simulink model "rotation"  (Simulink 7.0)
settings: Solver=ode45  SolverMode=SingleTasking  StartTime=0.0  StopTime=inf  RelTol=1e-3
values from neighbouring files (symbols this model uses):
  blk = 10    [rotation_init.m]
  col_delx_ws = ceil(col_delx*2^20)    [rotation_init.m]
  col_dely_ws = ceil(col_dely*2^20)    [rotation_init.m]
  fps = 1/(rows*(cols+3*blk))    [rotation_init.m]
  row_delx_ws = ceil(row_delx*2^20)*2    [rotation_init.m]
  row_dely_ws = ceil(row_dely*2^20)*2    [rotation_init.m]
  xstart_init_ws = ceil(xstart_init*2^20)    [rotation_init.m]
  ystart_init_ws = ceil(ystart_init*2^20)    [rotation_init.m]
undefined symbols (not defined in the file or in its folder): cols, rows
libraries: xbsIndex_r4 x273, dspsrcs4 x2, dspsigops x1, vipsrcs x1
(part 2 of 2)

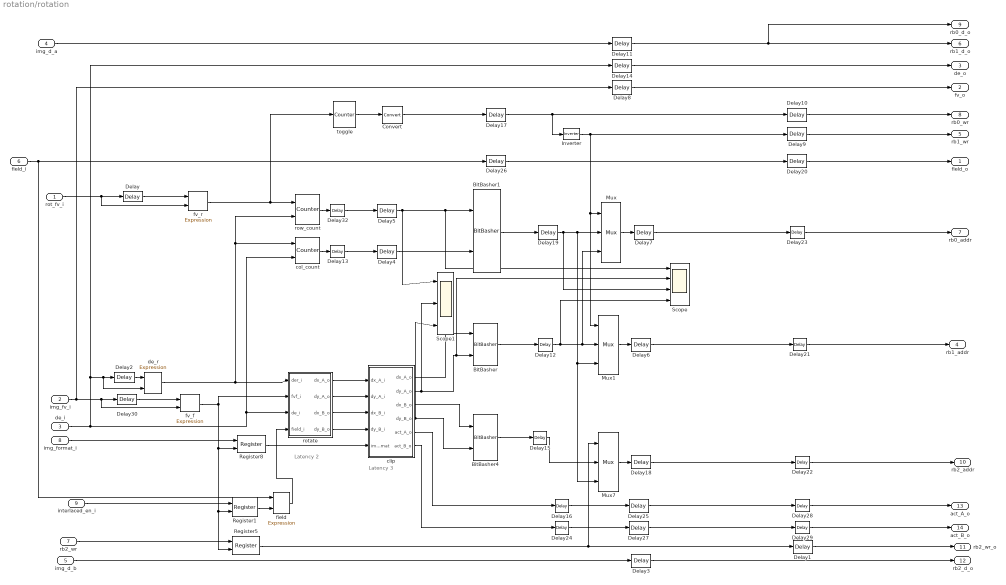
== system rotation/rotation ==
  note: Latency 3
  note: Latency 2
  rot_fv_i : Inport
  img_fv_i : Inport  Port=2
  de_i : Inport  Port=3
  img_d_a : Inport  Port=4
  img_d_b : Inport  Port=5
  field_i : Inport  Port=6
  rb2_wr : Inport  Port=7
  img_format_i : Inport  Port=8
  interlaced_en_i : Inport  Port=9
  BitBasher : xbsIndex_r4/BitBasher  bitexpr=|  display_expr=off  sr_1=1  arith_type1=Unsigned  bin_pt1=0  sr_2=2  arith_type2=Unsigned  bin_pt2=0  sr_3=3  arith_type3=Unsigned  bin_pt3=0  sr_4=4  arith_type4=Unsigned  bin_pt4=0  dbl_ovrd=off  block_type=bitbasher
      | <html><head><meta name="qrichtext" content="1" /><style type="text/css">
      | p, li { white-space: pre-wrap; }
      | </style></head><body style=" font-family:'MS Shell Dlg 2'; font-size:8.25pt; font-weight:400; font-style:normal;">
      | <p style=" margin-top:12px; margin-bottom:12px; margin-left:0px; margin-right:0px; -qt-block-indent:0; text-indent:0px; font-family:'MS Shell Dlg'; font-size:8pt;">addr={dy,dx}<br /></p></body></html>
      settings: block_version=10.1.3
  BitBasher1 : xbsIndex_r4/BitBasher  bitexpr=|  display_expr=off  sr_1=1  arith_type1=Unsigned  bin_pt1=0  sr_2=2  arith_type2=Unsigned  bin_pt2=0  sr_3=3  arith_type3=Unsigned  bin_pt3=0  sr_4=4  arith_type4=Unsigned  bin_pt4=0  dbl_ovrd=off  block_type=bitbasher
      | <html><head><meta name="qrichtext" content="1" /><style type="text/css">
      | p, li { white-space: pre-wrap; }
      | </style></head><body style=" font-family:'MS Shell Dlg 2'; font-size:8.25pt; font-weight:400; font-style:normal;">
      | <p style=" margin-top:12px; margin-bottom:12px; margin-left:0px; margin-right:0px; -qt-block-indent:0; text-indent:0px; font-family:'MS Shell Dlg'; font-size:8pt;">a={b,c}</p></body></html>
      settings: block_version=10.1.3
  BitBasher4 : xbsIndex_r4/BitBasher  bitexpr=|  display_expr=off  sr_1=1  arith_type1=Unsigned  bin_pt1=0  sr_2=2  arith_type2=Unsigned  bin_pt2=0  sr_3=3  arith_type3=Unsigned  bin_pt3=0  sr_4=4  arith_type4=Unsigned  bin_pt4=0  dbl_ovrd=off  block_type=bitbasher
      | <html><head><meta name="qrichtext" content="1" /><style type="text/css">
      | p, li { white-space: pre-wrap; }
      | </style></head><body style=" font-family:'MS Shell Dlg 2'; font-size:8.25pt; font-weight:400; font-style:normal;">
      | <p style=" margin-top:12px; margin-bottom:12px; margin-left:0px; margin-right:0px; -qt-block-indent:0; text-indent:0px; font-family:'MS Shell Dlg'; font-size:8pt;">addr={dy,dx}<br /></p></body></html>
      settings: block_version=10.1.3
  Convert : xbsIndex_r4/Convert  arith_type=Boolean  n_bits=16  bin_pt=14  quantization=Truncate  overflow=Wrap  latency=0  dbl_ovrd=off  pipeline=off  block_type=convert
      settings: block_version=10.1.3
  Delay{,1..2,6..7,12..13,15..16,18..19,21..25,27..30,32} (21 alike) : xbsIndex_r4/Delay  en=off  latency=1  dbl_ovrd=off  reg_retiming=off  block_type=delay
  Delay10 : xbsIndex_r4/Delay  en=off  latency=2  dbl_ovrd=off  reg_retiming=off  block_type=delay
  Delay{3,8,11,14} (4 alike) : xbsIndex_r4/Delay  en=off  latency=8  dbl_ovrd=off  reg_retiming=off  block_type=delay
  Delay17 : xbsIndex_r4/Delay  en=off  latency=5  dbl_ovrd=off  reg_retiming=off  block_type=delay
  Delay20 : xbsIndex_r4/Delay  en=off  latency=2  dbl_ovrd=off  reg_retiming=off  block_type=delay
  Delay26 : xbsIndex_r4/Delay  en=off  latency=5  dbl_ovrd=off  reg_retiming=off  block_type=delay
  Delay4 : xbsIndex_r4/Delay  en=off  latency=3  dbl_ovrd=off  reg_retiming=off  block_type=delay
  Delay5 : xbsIndex_r4/Delay  en=off  latency=3  dbl_ovrd=off  reg_retiming=off  block_type=delay
  Delay9 : xbsIndex_r4/Delay  en=off  latency=2  dbl_ovrd=off  reg_retiming=off  block_type=delay
  Inverter : xbsIndex_r4/Inverter  en=off  latency=0  dbl_ovrd=off  block_type=inv
  Mux : xbsIndex_r4/Mux  inputs=2  en=off  latency=0  precision=Full  arith_type=Unsigned  n_bits=16  bin_pt=14  quantization=Truncate  overflow=Wrap  dbl_ovrd=off  block_type=mux
  Mux1 : xbsIndex_r4/Mux  inputs=2  en=off  latency=0  precision=Full  arith_type=Unsigned  n_bits=16  bin_pt=14  quantization=Truncate  overflow=Wrap  dbl_ovrd=off  block_type=mux
  Mux7 : xbsIndex_r4/Mux  inputs=2  en=off  latency=0  precision=Full  arith_type=Unsigned  n_bits=16  bin_pt=14  quantization=Truncate  overflow=Wrap  dbl_ovrd=off  block_type=mux
  Register1 : xbsIndex_r4/Register  init=1  rst=off  en=on  dbl_ovrd=off  block_type=register
  Register5 : xbsIndex_r4/Register  init=1  rst=off  en=on  dbl_ovrd=off  block_type=register
  Register8 : xbsIndex_r4/Register  init=5  rst=off  en=on  dbl_ovrd=off  block_type=register
  Scope : Scope  NumInputPorts=4
      settings: TimeRange=100000  YMin=47.5~95~-1~-1  YMax=82.5~165~1~1
  Scope1 : Scope  NumInputPorts=3
      settings: TimeRange=150000  YMin=0~0~0  YMax=130~275~275
  clip : Subsystem
  col_count : xbsIndex_r4/Counter  cnt_type=Free Running  cnt_to=Inf  operation=Up  start_count=0  cnt_by_val=1  arith_type=Unsigned  n_bits=10  bin_pt=0  load_pin=off  rst=on  en=on  explicit_period=on  period=(1/fps)/ (rows*(cols+2*blk))  dbl_ovrd=off  use_behavioral_HDL=off  use_rpm=off  implementation=Fabric  block_type=counter
  de_r : xbsIndex_r4/Expression  expression=~a & b  align_bp=on  en=off  latency=0  precision=Full  arith_type=Unsigned  n_bits=16  bin_pt=0  dbl_ovrd=off  block_type=expr
      settings: block_version=10.1.3
  field : xbsIndex_r4/Expression  expression=a & b  align_bp=on  en=off  latency=0  precision=Full  arith_type=Unsigned  n_bits=16  bin_pt=0  dbl_ovrd=off  block_type=expr
      settings: block_version=10.1.3
  fv_f : xbsIndex_r4/Expression  expression=a & ~b  align_bp=on  en=off  latency=0  precision=Full  arith_type=Unsigned  n_bits=16  bin_pt=0  dbl_ovrd=off  block_type=expr
      settings: block_version=10.1.3
  fv_r : xbsIndex_r4/Expression  expression=~a &b  align_bp=on  en=off  latency=0  precision=Full  arith_type=Unsigned  n_bits=16  bin_pt=0  dbl_ovrd=off  block_type=expr
      settings: block_version=10.1.3
  rotate : Subsystem
  row_count : xbsIndex_r4/Counter  cnt_type=Free Running  cnt_to=Inf  operation=Up  start_count=0  cnt_by_val=1  arith_type=Unsigned  n_bits=10  bin_pt=0  load_pin=off  rst=on  en=on  explicit_period=on  period=(1/fps)/ (rows*(cols+2*blk))  dbl_ovrd=off  use_behavioral_HDL=off  use_rpm=off  implementation=Fabric  block_type=counter
  toggle : xbsIndex_r4/Counter  cnt_type=Free Running  cnt_to=Inf  operation=Up  start_count=1  cnt_by_val=1  arith_type=Unsigned  n_bits=1  bin_pt=0  load_pin=off  rst=off  en=on  explicit_period=on  period=(1/fps)/ (rows*(cols+2*blk))  dbl_ovrd=off  use_behavioral_HDL=off  use_rpm=off  implementation=Fabric  block_type=counter
  field_o : Outport
  fv_o : Outport  Port=2
  de_o : Outport  Port=3
  rb1_addr : Outport  Port=4
  rb1_wr : Outport  Port=5
  rb1_d_o : Outport  Port=6
  rb0_addr : Outport  Port=7
  rb0_wr : Outport  Port=8
  rb0_d_o : Outport  Port=9
  rb2_addr : Outport  Port=10
  rb2_wr_o : Outport  Port=11
  rb2_d_o : Outport  Port=12
  act_A_o : Outport  Port=13
  act_B_o : Outport  Port=14
  wires:
  rotate/2(dy_A_o) -> clip/2(dy_A_i)
  rotate/1(dx_A_o) -> clip/1(dx_A_i)
  fv_r/1 -> row_count/1, toggle/1
  Delay2/1 -> de_r/1
  Delay/1 -> fv_r/1
  img_d_a/1 -> Delay11/1
  Delay8/1 -> fv_o/1
  Delay14/1 -> de_o/1
  de_r/1 -> rotate/1(der_i), col_count/1, row_count/2
  col_count/1 -> Delay13/1
  Mux1/1 -> Delay6/1
  Mux/1 -> Delay7/1
  toggle/1 -> Convert/1
  Inverter/1 -> Mux/1, Mux1/1, Delay9/1
  Delay11/1 -> rb1_d_o/1, rb0_d_o/1
  Convert/1 -> Delay17/1
  Delay9/1 -> rb1_wr/1
  Delay10/1 -> rb0_wr/1
  Delay17/1 -> Inverter/1, Delay10/1
  rotate/3(dx_B_o) -> clip/3(dx_B_i)
  rotate/4(dy_B_o) -> clip/4(dy_B_i)
  row_count/1 -> Delay32/1
  de_i/1 -> rotate/3(de_i), col_count/2, Delay14/1, Delay2/1, de_r/2
  img_d_b/1 -> Delay3/1
  Delay3/1 -> rb2_d_o/1
  Delay26/1 -> Delay20/1
  Delay20/1 -> field_o/1
  Mux7/1 -> Delay18/1
  Register5/1 -> Mux7/1, Delay1/1
  Delay7/1 -> Delay23/1
  Delay1/1 -> rb2_wr_o/1
  field_i/1 -> Delay26/1, field/1
  img_format_i/1 -> Register8/1
  BitBasher1/1 -> Delay19/1
  Register8/1 -> clip/5(img_format)
  rot_fv_i/1 -> Delay/1, fv_r/2
  fv_f/1 -> Register8/2, Register5/2, Register1/2, rotate/2(fvf_i)
  Delay19/1 -> Mux/2, Mux1/3, Mux7/3, Scope/3
  BitBasher/1 -> Delay12/1
  Delay5/1 -> BitBasher1/1, Scope/1, Scope1/1
  Delay4/1 -> BitBasher1/2
  Delay23/1 -> rb0_addr/1
  Delay21/1 -> rb1_addr/1
  Delay22/1 -> rb2_addr/1
  Delay12/1 -> Mux/3, Mux1/2, Scope/4
  BitBasher4/1 -> Delay15/1
  Delay15/1 -> Mux7/2
  rb2_wr/1 -> Register5/1
  clip/1(dx_A_o) -> BitBasher/1
  clip/2(dy_A_o) -> BitBasher/2, Scope/2, Scope1/2
  clip/3(dx_B_o) -> BitBasher4/1
  clip/4(dy_B_o) -> BitBasher4/2, Scope1/3
  clip/5(act_A_o) -> Delay16/1
  clip/6(act_B_o) -> Delay24/1
  Delay16/1 -> Delay25/1
  Delay24/1 -> Delay27/1
  Delay25/1 -> Delay28/1
  Delay27/1 -> Delay29/1
  Delay28/1 -> act_A_o/1
  Delay29/1 -> act_B_o/1
  Delay6/1 -> Delay21/1
  Delay18/1 -> Delay22/1
  img_fv_i/1 -> Delay30/1, fv_f/2, Delay8/1
  Delay30/1 -> fv_f/1
  interlaced_en_i/1 -> Register1/1
  Register1/1 -> field/2
  field/1 -> rotate/4(field_i)
  Delay13/1 -> Delay4/1
  Delay32/1 -> Delay5/1

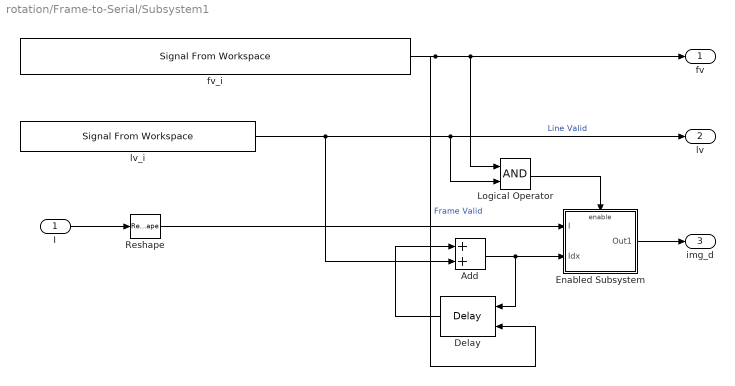
== system rotation/Frame-to-Serial/Subsystem1 ==
  I : Inport  OutDataType=sfix(16)  OutScaling=2^0
  Add : Sum  OutDataType=sfix(16)  OutScaling=2^-10
  Delay : dspsigops/Delay  Orientation=left  dly_unit=Samples  delay=1  ic_detail=off  dif_ic_for_ch=off  dif_ic_for_dly=off  ic=0  reset_popup=Falling edge
  Enabled Subsystem : Subsystem  TreatAsAtomicUnit=on
  Logical Operator : Logic  AllPortsSameDT=off  OutDataTypeMode=boolean
  Reshape : Reshape
  fv_i : dspsrcs4/Signal From Workspace  SystemSampleTime=-1  X=[ zeros(1,blk) ones(1,rows*(cols+2*blk)-2*blk) zeros(1,blk) ]  Ts=(1/fps)/(rows*(cols+2*blk))  nsamps=1  OutputAfterFinalValue=Cyclic repetition  ignoreOrWarnInputAndFrameLengths=off
  lv_i : dspsrcs4/Signal From Workspace  SystemSampleTime=-1  X=[zeros(1,blk) ones(1,cols) zeros(1,blk)]  Ts=(1/fps)/ (rows*(cols+2*blk))  nsamps=1  OutputAfterFinalValue=Cyclic repetition  ignoreOrWarnInputAndFrameLengths=off
  fv : Outport  OutDataType=sfix(16)  OutScaling=2^0
  lv : Outport  Port=2  OutDataType=sfix(16)  OutScaling=2^0
  img_d : Outport  Port=3  OutDataType=sfix(16)  OutScaling=2^0
  wires:
  I/1 -> Reshape/1
  fv_i/1 -> Delay/2, fv/1, Logical Operator/1  "Frame Valid"
  lv_i/1 -> Add/2, lv/1, Logical Operator/2  "Line Valid"
  Delay/1 -> Add/1
  Add/1 -> Delay/1, Enabled Subsystem/2(Idx)
  Enabled Subsystem/1(Out1) -> img_d/1
  Reshape/1 -> Enabled Subsystem/1(I)
  Logical Operator/1 -> Enabled Subsystem/Enable

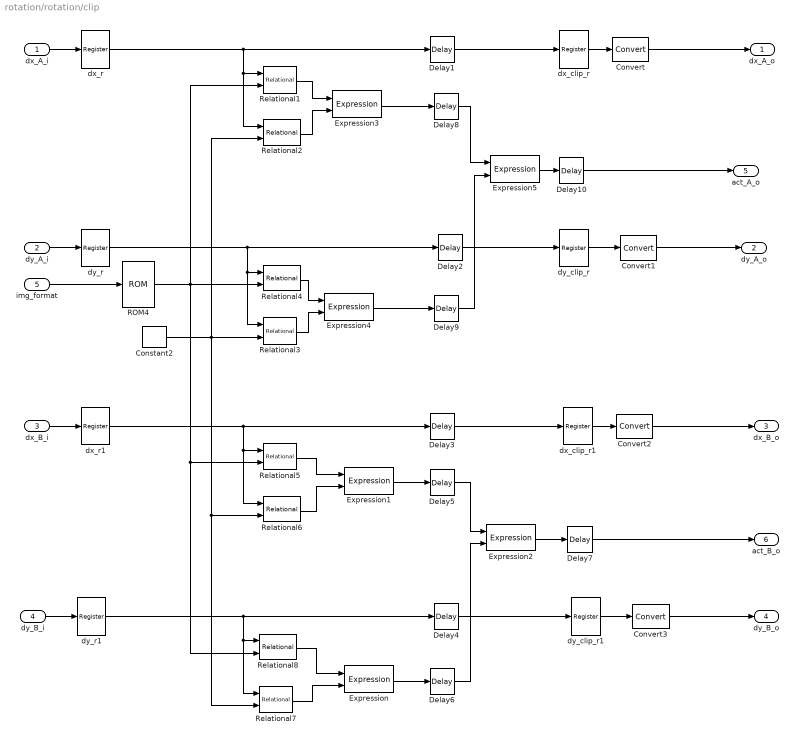
== system rotation/rotation/clip ==
  dx_A_i : Inport
  dy_A_i : Inport  Port=2
  dx_B_i : Inport  Port=3
  dy_B_i : Inport  Port=4
  img_format : Inport  Port=5
  Constant2 : xbsIndex_r4/Constant  arith_type=Signed (2's comp)  const=0  n_bits=11  bin_pt=0  explicit_period=on  period=(1/fps)/ (rows*(cols+2*blk))  equ=P=C  opselect=C  inp2=PCIN>>17  opr=+  inp1=P  carry=CIN  dbl_ovrd=off  block_type=constant
  Convert{,1..3} (4 alike) : xbsIndex_r4/Convert  arith_type=Unsigned  n_bits=10  bin_pt=0  quantization=Truncate  overflow=Wrap  latency=0  dbl_ovrd=off  pipeline=off  block_type=convert
      settings: block_version=10.1.3
  Delay{1..10} (10 alike) : xbsIndex_r4/Delay  en=off  latency=1  dbl_ovrd=off  reg_retiming=off  block_type=delay
  Expression{,1,3..4} (4 alike) : xbsIndex_r4/Expression  expression=a | b  align_bp=on  en=off  latency=0  precision=Full  arith_type=Unsigned  n_bits=16  bin_pt=0  dbl_ovrd=off  block_type=expr
      settings: block_version=10.1.3
  Expression2 : xbsIndex_r4/Expression  expression=~(a | b)  align_bp=on  en=off  latency=0  precision=Full  arith_type=Unsigned  n_bits=16  bin_pt=0  dbl_ovrd=off  block_type=expr
      settings: block_version=10.1.3
  Expression5 : xbsIndex_r4/Expression  expression=~(a | b)  align_bp=on  en=off  latency=0  precision=Full  arith_type=Unsigned  n_bits=16  bin_pt=0  dbl_ovrd=off  block_type=expr
      settings: block_version=10.1.3
  ROM4 : xbsIndex_r4/ROM  depth=8  initVector=[479 599 767 479 575 1023 0 0 0]  distributed_mem=Distributed memory  rst=off  init_reg=0  en=off  latency=1  arith_type="Signed  (2's comp)"  n_bits=11  bin_pt=0  dbl_ovrd=off  optimize=Area  use_rpm=on  block_type=sprom
      settings: block_version=10.1.3
  Relational{1,4..5,8} (4 alike) : xbsIndex_r4/Relational  mode=a>b  en=off  latency=0  dbl_ovrd=off  block_type=relational
      settings: block_version=10.1.3
  Relational{2..3,6..7} (4 alike) : xbsIndex_r4/Relational  mode=a<b  en=off  latency=0  dbl_ovrd=off  block_type=relational
      settings: block_version=10.1.3
  dx_clip_r : xbsIndex_r4/Register  init=0  rst=off  en=off  dbl_ovrd=off  block_type=register
  dx_clip_r1 : xbsIndex_r4/Register  init=0  rst=off  en=off  dbl_ovrd=off  block_type=register
  dx_r : xbsIndex_r4/Register  init=0  rst=off  en=off  dbl_ovrd=off  block_type=register
  dx_r1 : xbsIndex_r4/Register  init=0  rst=off  en=off  dbl_ovrd=off  block_type=register
  dy_clip_r : xbsIndex_r4/Register  init=0  rst=off  en=off  dbl_ovrd=off  block_type=register
  dy_clip_r1 : xbsIndex_r4/Register  init=0  rst=off  en=off  dbl_ovrd=off  block_type=register
  dy_r : xbsIndex_r4/Register  init=0  rst=off  en=off  dbl_ovrd=off  block_type=register
  dy_r1 : xbsIndex_r4/Register  init=0  rst=off  en=off  dbl_ovrd=off  block_type=register
  dx_A_o : Outport  OutDataType=sfix(16)  OutScaling=2^0
  dy_A_o : Outport  Port=2  OutDataType=sfix(16)  OutScaling=2^0
  dx_B_o : Outport  Port=3  OutDataType=sfix(16)  OutScaling=2^0
  dy_B_o : Outport  Port=4  OutDataType=sfix(16)  OutScaling=2^0
  act_A_o : Outport  Port=5  OutDataType=sfix(16)  OutScaling=2^0
  act_B_o : Outport  Port=6  OutDataType=sfix(16)  OutScaling=2^0
  wires:
  dx_A_i/1 -> dx_r/1
  dx_r/1 -> Relational2/1, Relational1/1, Delay1/1
  dy_A_i/1 -> dy_r/1
  dy_r/1 -> Relational3/1, Relational4/1, Delay2/1
  Constant2/1 -> Relational3/2, Relational2/2, Relational7/2, Relational6/2
  ROM4/1 -> Relational4/2, Relational5/2, Relational8/2, Relational1/2
  dx_clip_r/1 -> Convert/1
  Convert/1 -> dx_A_o/1
  dy_clip_r/1 -> Convert1/1
  Convert1/1 -> dy_A_o/1
  dx_B_i/1 -> dx_r1/1
  dx_r1/1 -> Relational6/1, Relational5/1, Delay3/1
  dy_B_i/1 -> dy_r1/1
  dy_r1/1 -> Relational7/1, Relational8/1, Delay4/1
  dx_clip_r1/1 -> Convert2/1
  Convert2/1 -> dx_B_o/1
  dy_clip_r1/1 -> Convert3/1
  Convert3/1 -> dy_B_o/1
  img_format/1 -> ROM4/1
  Delay1/1 -> dx_clip_r/1
  Delay2/1 -> dy_clip_r/1
  Delay3/1 -> dx_clip_r1/1
  Delay4/1 -> dy_clip_r1/1
  Relational8/1 -> Expression/1
  Relational7/1 -> Expression/2
  Relational5/1 -> Expression1/1
  Relational6/1 -> Expression1/2
  Expression1/1 -> Delay5/1
  Expression/1 -> Delay6/1
  Delay5/1 -> Expression2/1
  Delay6/1 -> Expression2/2
  Expression2/1 -> Delay7/1
  Delay7/1 -> act_B_o/1
  Relational1/1 -> Expression3/1
  Relational2/1 -> Expression3/2
  Expression3/1 -> Delay8/1
  Relational4/1 -> Expression4/1
  Relational3/1 -> Expression4/2
  Expression4/1 -> Delay9/1
  Delay8/1 -> Expression5/1
  Delay9/1 -> Expression5/2
  Expression5/1 -> Delay10/1
  Delay10/1 -> act_A_o/1

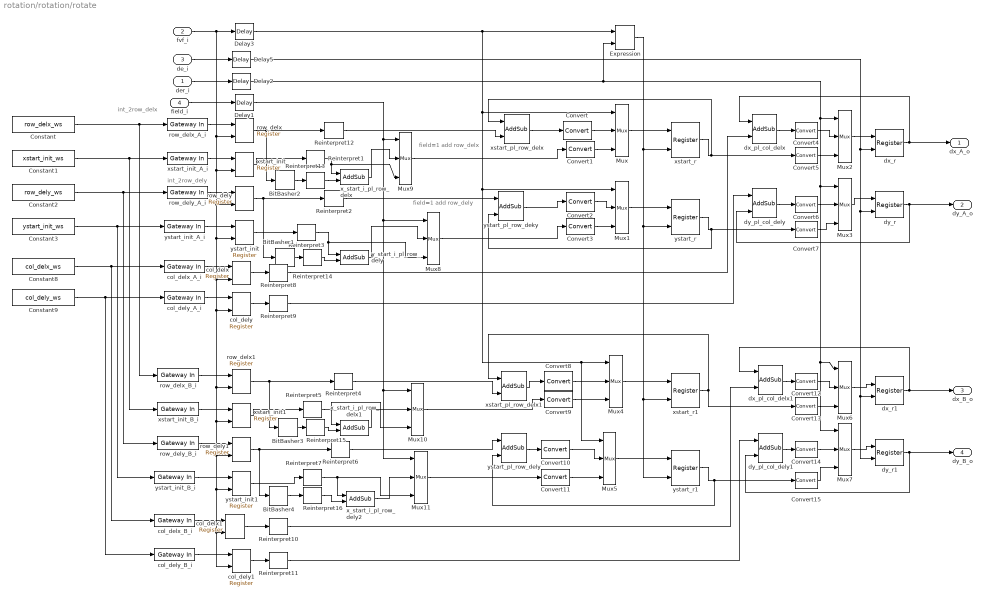
== system rotation/rotation/rotate ==
  note: int_2row_dely
  note: field=1 add row_delx
  note: field=1 add row_dely
  note: int_2row_delx
  der_i : Inport
  fvf_i : Inport  Port=2
  de_i : Inport  Port=3
  field_i : Inport  Port=4
  BitBasher1 : xbsIndex_r4/BitBasher  bitexpr=|  display_expr=off  sr_1=1  arith_type1="Signed  (2's comp)"  bin_pt1=0  sr_2=2  arith_type2=Unsigned  bin_pt2=0  sr_3=3  arith_type3=Unsigned  bin_pt3=0  sr_4=4  arith_type4=Unsigned  bin_pt4=0  dbl_ovrd=off  block_type=bitbasher
      | <html><head><meta name="qrichtext" content="1" /><style type="text/css">
      | p, li { white-space: pre-wrap; }
      | </style></head><body style=" font-family:'MS Shell Dlg 2'; font-size:8.25pt; font-weight:400; font-style:normal;">
      | <p style=" margin-top:12px; margin-bottom:12px; margin-left:0px; margin-right:0px; -qt-block-indent:0; text-indent:0px; font-family:'MS Shell Dlg'; font-size:8pt;">b={a[31],a[31:1]}<br /></p></body></html>
      settings: block_version=10.1.3
  BitBasher2 : xbsIndex_r4/BitBasher  bitexpr=|  display_expr=off  sr_1=1  arith_type1="Signed  (2's comp)"  bin_pt1=0  sr_2=2  arith_type2=Unsigned  bin_pt2=0  sr_3=3  arith_type3=Unsigned  bin_pt3=0  sr_4=4  arith_type4=Unsigned  bin_pt4=0  dbl_ovrd=off  block_type=bitbasher
      | <html><head><meta name="qrichtext" content="1" /><style type="text/css">
      | p, li { white-space: pre-wrap; }
      | </style></head><body style=" font-family:'MS Shell Dlg 2'; font-size:8.25pt; font-weight:400; font-style:normal;">
      | <p style=" margin-top:12px; margin-bottom:12px; margin-left:0px; margin-right:0px; -qt-block-indent:0; text-indent:0px; font-family:'MS Shell Dlg'; font-size:8pt;">b={a[31],a[31:1]}<br /></p></body></html>
      settings: block_version=10.1.3
  BitBasher3 : xbsIndex_r4/BitBasher  bitexpr=|  display_expr=off  sr_1=1  arith_type1="Signed  (2's comp)"  bin_pt1=0  sr_2=2  arith_type2=Unsigned  bin_pt2=0  sr_3=3  arith_type3=Unsigned  bin_pt3=0  sr_4=4  arith_type4=Unsigned  bin_pt4=0  dbl_ovrd=off  block_type=bitbasher
      | <html><head><meta name="qrichtext" content="1" /><style type="text/css">
      | p, li { white-space: pre-wrap; }
      | </style></head><body style=" font-family:'MS Shell Dlg 2'; font-size:8.25pt; font-weight:400; font-style:normal;">
      | <p style=" margin-top:12px; margin-bottom:12px; margin-left:0px; margin-right:0px; -qt-block-indent:0; text-indent:0px; font-family:'MS Shell Dlg'; font-size:8pt;">b={a[31],a[31:1]}<br /></p></body></html>
      settings: block_version=10.1.3
  BitBasher4 : xbsIndex_r4/BitBasher  bitexpr=|  display_expr=off  sr_1=1  arith_type1="Signed  (2's comp)"  bin_pt1=0  sr_2=2  arith_type2=Unsigned  bin_pt2=0  sr_3=3  arith_type3=Unsigned  bin_pt3=0  sr_4=4  arith_type4=Unsigned  bin_pt4=0  dbl_ovrd=off  block_type=bitbasher
      | <html><head><meta name="qrichtext" content="1" /><style type="text/css">
      | p, li { white-space: pre-wrap; }
      | </style></head><body style=" font-family:'MS Shell Dlg 2'; font-size:8.25pt; font-weight:400; font-style:normal;">
      | <p style=" margin-top:12px; margin-bottom:12px; margin-left:0px; margin-right:0px; -qt-block-indent:0; text-indent:0px; font-family:'MS Shell Dlg'; font-size:8pt;">b={a[31],a[31:1]}<br /></p></body></html>
      settings: block_version=10.1.3
  Constant : Constant  Value=row_delx_ws  OutDataType=sfix(16)  OutScaling=2^0
  Constant1 : Constant  Value=xstart_init_ws  OutDataType=sfix(16)  OutScaling=2^0
  Constant2 : Constant  Value=row_dely_ws  OutDataType=sfix(16)  OutScaling=2^0
  Constant3 : Constant  Value=ystart_init_ws  OutDataType=sfix(16)  OutScaling=2^0
  Constant8 : Constant  Value=col_delx_ws  OutDataType=sfix(16)  OutScaling=2^0
  Constant9 : Constant  Value=col_dely_ws  OutDataType=sfix(16)  OutScaling=2^0
  Convert{,1..15} (16 alike) : xbsIndex_r4/Convert  arith_type="Signed  (2's comp)"  n_bits=32  bin_pt=20  quantization=Truncate  overflow=Wrap  latency=0  dbl_ovrd=off  pipeline=off  block_type=convert
      settings: block_version=10.1.3
  Delay{1..3,5} (4 alike) : xbsIndex_r4/Delay  en=off  latency=1  dbl_ovrd=off  reg_retiming=off  block_type=delay
  Expression : xbsIndex_r4/Expression  expression=a | b  align_bp=on  en=off  latency=0  precision=Full  arith_type=Unsigned  n_bits=16  bin_pt=0  dbl_ovrd=off  block_type=expr
      settings: block_version=10.1.3
  Mux{,1..11} (12 alike) : xbsIndex_r4/Mux  inputs=2  en=off  latency=0  precision=Full  arith_type=Unsigned  n_bits=16  bin_pt=14  quantization=Truncate  overflow=Wrap  dbl_ovrd=off  block_type=mux
  Reinterpret{1..16} (16 alike) : xbsIndex_r4/Reinterpret  force_arith_type=on  arith_type="Signed  (2's comp)"  force_bin_pt=on  bin_pt=20  block_type=reinterpret
      settings: infoedit="Changes signal type without altering the binary representation.   You can changed the signal between signed and unsigned, and relocate the binary point.<P><P>Hardware notes: In hardware this block costs nothing.<P><P>Example:  Suppose the input is 6 bits wide, signed, with 2 fractional bits, and the output is forced to unsigned with 0 fractional bits.  Then an input of -2.0 (1110.00 in binary 2's complement) becomes an output of 56 (111000 in binary)."  block_version=10.1.3
  col_delx : xbsIndex_r4/Register  init=col_delx_ws  rst=off  en=on  dbl_ovrd=off  block_type=register
  col_delx1 : xbsIndex_r4/Register  init=col_delx_ws  rst=off  en=on  dbl_ovrd=off  block_type=register
  col_delx_A_i : xbsIndex_r4/Gateway In  arith_type="Signed  (2's comp)"  n_bits=32  bin_pt=0  quantization=Truncate  overflow=Wrap  period=(1/fps)/ (rows*(cols+2*blk))  dbl_ovrd=off  timing_constraint=None  locs_specified=off  LOCs={}  block_type=gatewayin
      settings: infoedit="Gateway in block.  Converts inputs of type Simulink integer, double and fixed point to  Xilinx fixed point type.<P><P>Hardware notes:  In hardware these blocks become top level input ports."  block_version=10.1.3
  col_delx_B_i : xbsIndex_r4/Gateway In  arith_type="Signed  (2's comp)"  n_bits=32  bin_pt=0  quantization=Truncate  overflow=Wrap  period=(1/fps)/ (rows*(cols+2*blk))  dbl_ovrd=off  timing_constraint=None  locs_specified=off  LOCs={}  block_type=gatewayin
      settings: infoedit="Gateway in block.  Converts inputs of type Simulink integer, double and fixed point to  Xilinx fixed point type.<P><P>Hardware notes:  In hardware these blocks become top level input ports."  block_version=10.1.3
  col_dely : xbsIndex_r4/Register  init=col_dely_ws  rst=off  en=on  dbl_ovrd=off  block_type=register
  col_dely1 : xbsIndex_r4/Register  init=col_dely_ws  rst=off  en=on  dbl_ovrd=off  block_type=register
  col_dely_A_i : xbsIndex_r4/Gateway In  arith_type="Signed  (2's comp)"  n_bits=32  bin_pt=0  quantization=Truncate  overflow=Wrap  period=(1/fps)/ (rows*(cols+2*blk))  dbl_ovrd=off  timing_constraint=None  locs_specified=off  LOCs={}  block_type=gatewayin
      settings: infoedit="Gateway in block.  Converts inputs of type Simulink integer, double and fixed point to  Xilinx fixed point type.<P><P>Hardware notes:  In hardware these blocks become top level input ports."  block_version=10.1.3
  col_dely_B_i : xbsIndex_r4/Gateway In  arith_type="Signed  (2's comp)"  n_bits=32  bin_pt=0  quantization=Truncate  overflow=Wrap  period=(1/fps)/ (rows*(cols+2*blk))  dbl_ovrd=off  timing_constraint=None  locs_specified=off  LOCs={}  block_type=gatewayin
      settings: infoedit="Gateway in block.  Converts inputs of type Simulink integer, double and fixed point to  Xilinx fixed point type.<P><P>Hardware notes:  In hardware these blocks become top level input ports."  block_version=10.1.3
  dx_pl_col_delx : xbsIndex_r4/AddSub  mode=Addition  use_carryin=off  use_carryout=off  en=off  latency=0  precision=Full  arith_type=Unsigned  n_bits=16  bin_pt=14  quantization=Truncate  overflow=Wrap  dbl_ovrd=off  use_behavioral_HDL=off  pipelined=off  use_rpm=on  hw_selection=Fabric  block_type=addsub
      settings: block_version=10.1.3
  dx_pl_col_delx1 : xbsIndex_r4/AddSub  mode=Addition  use_carryin=off  use_carryout=off  en=off  latency=0  precision=Full  arith_type=Unsigned  n_bits=16  bin_pt=14  quantization=Truncate  overflow=Wrap  dbl_ovrd=off  use_behavioral_HDL=off  pipelined=off  use_rpm=on  hw_selection=Fabric  block_type=addsub
      settings: block_version=10.1.3
  dx_r : xbsIndex_r4/Register  init=col_delx_ws/2^20  rst=off  en=on  dbl_ovrd=off  block_type=register
  dx_r1 : xbsIndex_r4/Register  init=col_delx_ws/2^20  rst=off  en=on  dbl_ovrd=off  block_type=register
  dy_pl_col_dely : xbsIndex_r4/AddSub  mode=Addition  use_carryin=off  use_carryout=off  en=off  latency=0  precision=Full  arith_type=Unsigned  n_bits=16  bin_pt=14  quantization=Truncate  overflow=Wrap  dbl_ovrd=off  use_behavioral_HDL=off  pipelined=off  use_rpm=on  hw_selection=Fabric  block_type=addsub
      settings: block_version=10.1.3
  dy_pl_col_dely1 : xbsIndex_r4/AddSub  mode=Addition  use_carryin=off  use_carryout=off  en=off  latency=0  precision=Full  arith_type=Unsigned  n_bits=16  bin_pt=14  quantization=Truncate  overflow=Wrap  dbl_ovrd=off  use_behavioral_HDL=off  pipelined=off  use_rpm=on  hw_selection=Fabric  block_type=addsub
      settings: block_version=10.1.3
  dy_r : xbsIndex_r4/Register  init=col_dely_ws/2^20  rst=off  en=on  dbl_ovrd=off  block_type=register
  dy_r1 : xbsIndex_r4/Register  init=col_dely_ws/2^20  rst=off  en=on  dbl_ovrd=off  block_type=register
  row_delx : xbsIndex_r4/Register  init=row_delx_ws  rst=off  en=on  dbl_ovrd=off  block_type=register
  row_delx1 : xbsIndex_r4/Register  init=row_delx_ws  rst=off  en=on  dbl_ovrd=off  block_type=register
  row_delx_A_i : xbsIndex_r4/Gateway In  arith_type="Signed  (2's comp)"  n_bits=32  bin_pt=0  quantization=Truncate  overflow=Wrap  period=(1/fps)/ (rows*(cols+2*blk))  dbl_ovrd=off  timing_constraint=None  locs_specified=off  LOCs={}  block_type=gatewayin
      settings: infoedit="Gateway in block.  Converts inputs of type Simulink integer, double and fixed point to  Xilinx fixed point type.<P><P>Hardware notes:  In hardware these blocks become top level input ports."  block_version=10.1.3
  row_delx_B_i : xbsIndex_r4/Gateway In  arith_type="Signed  (2's comp)"  n_bits=32  bin_pt=0  quantization=Truncate  overflow=Wrap  period=(1/fps)/ (rows*(cols+2*blk))  dbl_ovrd=off  timing_constraint=None  locs_specified=off  LOCs={}  block_type=gatewayin
      settings: infoedit="Gateway in block.  Converts inputs of type Simulink integer, double and fixed point to  Xilinx fixed point type.<P><P>Hardware notes:  In hardware these blocks become top level input ports."  block_version=10.1.3
  row_dely : xbsIndex_r4/Register  init=row_dely_ws  rst=off  en=on  dbl_ovrd=off  block_type=register
  row_dely1 : xbsIndex_r4/Register  init=row_dely_ws  rst=off  en=on  dbl_ovrd=off  block_type=register
  row_dely_A_i : xbsIndex_r4/Gateway In  arith_type="Signed  (2's comp)"  n_bits=32  bin_pt=0  quantization=Truncate  overflow=Wrap  period=(1/fps)/ (rows*(cols+2*blk))  dbl_ovrd=off  timing_constraint=None  locs_specified=off  LOCs={}  block_type=gatewayin
      settings: infoedit="Gateway in block.  Converts inputs of type Simulink integer, double and fixed point to  Xilinx fixed point type.<P><P>Hardware notes:  In hardware these blocks become top level input ports."  block_version=10.1.3
  row_dely_B_i : xbsIndex_r4/Gateway In  arith_type="Signed  (2's comp)"  n_bits=32  bin_pt=0  quantization=Truncate  overflow=Wrap  period=(1/fps)/ (rows*(cols+2*blk))  dbl_ovrd=off  timing_constraint=None  locs_specified=off  LOCs={}  block_type=gatewayin
      settings: infoedit="Gateway in block.  Converts inputs of type Simulink integer, double and fixed point to  Xilinx fixed point type.<P><P>Hardware notes:  In hardware these blocks become top level input ports."  block_version=10.1.3
  x_start_i_pl_row_delx : xbsIndex_r4/AddSub  mode=Addition  use_carryin=off  use_carryout=off  en=off  latency=0  precision=Full  arith_type=Unsigned  n_bits=16  bin_pt=14  quantization=Truncate  overflow=Wrap  dbl_ovrd=off  use_behavioral_HDL=off  pipelined=off  use_rpm=on  hw_selection=Fabric  block_type=addsub
      settings: block_version=10.1.3
  x_start_i_pl_row_delx1 : xbsIndex_r4/AddSub  mode=Addition  use_carryin=off  use_carryout=off  en=off  latency=0  precision=Full  arith_type=Unsigned  n_bits=16  bin_pt=14  quantization=Truncate  overflow=Wrap  dbl_ovrd=off  use_behavioral_HDL=off  pipelined=off  use_rpm=on  hw_selection=Fabric  block_type=addsub
      settings: block_version=10.1.3
  x_start_i_pl_row_dely2 : xbsIndex_r4/AddSub  mode=Addition  use_carryin=off  use_carryout=off  en=off  latency=0  precision=Full  arith_type=Unsigned  n_bits=16  bin_pt=14  quantization=Truncate  overflow=Wrap  dbl_ovrd=off  use_behavioral_HDL=off  pipelined=off  use_rpm=on  hw_selection=Fabric  block_type=addsub
      settings: block_version=10.1.3
  xstart_init : xbsIndex_r4/Register  init=xstart_init_ws  rst=off  en=on  dbl_ovrd=off  block_type=register
  xstart_init1 : xbsIndex_r4/Register  init=xstart_init_ws  rst=off  en=on  dbl_ovrd=off  block_type=register
  xstart_init_A_i : xbsIndex_r4/Gateway In  arith_type="Signed  (2's comp)"  n_bits=32  bin_pt=0  quantization=Truncate  overflow=Wrap  period=(1/fps)/ (rows*(cols+2*blk))  dbl_ovrd=off  timing_constraint=None  locs_specified=off  LOCs={}  block_type=gatewayin
      settings: infoedit="Gateway in block.  Converts inputs of type Simulink integer, double and fixed point to  Xilinx fixed point type.<P><P>Hardware notes:  In hardware these blocks become top level input ports."  block_version=10.1.3
  xstart_init_B_i : xbsIndex_r4/Gateway In  arith_type="Signed  (2's comp)"  n_bits=32  bin_pt=0  quantization=Truncate  overflow=Wrap  period=(1/fps)/ (rows*(cols+2*blk))  dbl_ovrd=off  timing_constraint=None  locs_specified=off  LOCs={}  block_type=gatewayin
      settings: infoedit="Gateway in block.  Converts inputs of type Simulink integer, double and fixed point to  Xilinx fixed point type.<P><P>Hardware notes:  In hardware these blocks become top level input ports."  block_version=10.1.3
  xstart_pl_row_delx : xbsIndex_r4/AddSub  mode=Addition  use_carryin=off  use_carryout=off  en=off  latency=0  precision=Full  arith_type=Unsigned  n_bits=16  bin_pt=14  quantization=Truncate  overflow=Wrap  dbl_ovrd=off  use_behavioral_HDL=off  pipelined=off  use_rpm=on  hw_selection=Fabric  block_type=addsub
      settings: block_version=10.1.3
  xstart_pl_row_delx1 : xbsIndex_r4/AddSub  mode=Addition  use_carryin=off  use_carryout=off  en=off  latency=0  precision=Full  arith_type=Unsigned  n_bits=16  bin_pt=14  quantization=Truncate  overflow=Wrap  dbl_ovrd=off  use_behavioral_HDL=off  pipelined=off  use_rpm=on  hw_selection=Fabric  block_type=addsub
      settings: block_version=10.1.3
  xstart_r : xbsIndex_r4/Register  init=xstart_init_ws/2^20  rst=off  en=on  dbl_ovrd=off  block_type=register
  xstart_r1 : xbsIndex_r4/Register  init=xstart_init_ws/2^20  rst=off  en=on  dbl_ovrd=off  block_type=register
  y_start_i_pl_row_dely : xbsIndex_r4/AddSub  mode=Addition  use_carryin=off  use_carryout=off  en=off  latency=0  precision=Full  arith_type=Unsigned  n_bits=16  bin_pt=14  quantization=Truncate  overflow=Wrap  dbl_ovrd=off  use_behavioral_HDL=off  pipelined=off  use_rpm=on  hw_selection=Fabric  block_type=addsub
      settings: block_version=10.1.3
  ystart_init : xbsIndex_r4/Register  init=ystart_init_ws  rst=off  en=on  dbl_ovrd=off  block_type=register
  ystart_init1 : xbsIndex_r4/Register  init=ystart_init_ws  rst=off  en=on  dbl_ovrd=off  block_type=register
  ystart_init_A_i : xbsIndex_r4/Gateway In  arith_type="Signed  (2's comp)"  n_bits=32  bin_pt=0  quantization=Truncate  overflow=Wrap  period=(1/fps)/ (rows*(cols+2*blk))  dbl_ovrd=off  timing_constraint=None  locs_specified=off  LOCs={}  block_type=gatewayin
      settings: infoedit="Gateway in block.  Converts inputs of type Simulink integer, double and fixed point to  Xilinx fixed point type.<P><P>Hardware notes:  In hardware these blocks become top level input ports."  block_version=10.1.3
  ystart_init_B_i : xbsIndex_r4/Gateway In  arith_type="Signed  (2's comp)"  n_bits=32  bin_pt=0  quantization=Truncate  overflow=Wrap  period=(1/fps)/ (rows*(cols+2*blk))  dbl_ovrd=off  timing_constraint=None  locs_specified=off  LOCs={}  block_type=gatewayin
      settings: infoedit="Gateway in block.  Converts inputs of type Simulink integer, double and fixed point to  Xilinx fixed point type.<P><P>Hardware notes:  In hardware these blocks become top level input ports."  block_version=10.1.3
  ystart_pl_row_deky : xbsIndex_r4/AddSub  mode=Addition  use_carryin=off  use_carryout=off  en=off  latency=0  precision=Full  arith_type=Unsigned  n_bits=16  bin_pt=14  quantization=Truncate  overflow=Wrap  dbl_ovrd=off  use_behavioral_HDL=off  pipelined=off  use_rpm=on  hw_selection=Fabric  block_type=addsub
      settings: block_version=10.1.3
  ystart_pl_row_dely : xbsIndex_r4/AddSub  mode=Addition  use_carryin=off  use_carryout=off  en=off  latency=0  precision=Full  arith_type=Unsigned  n_bits=16  bin_pt=14  quantization=Truncate  overflow=Wrap  dbl_ovrd=off  use_behavioral_HDL=off  pipelined=off  use_rpm=on  hw_selection=Fabric  block_type=addsub
      settings: block_version=10.1.3
  ystart_r : xbsIndex_r4/Register  init=ystart_init_ws/2^20  rst=off  en=on  dbl_ovrd=off  block_type=register
  ystart_r1 : xbsIndex_r4/Register  init=ystart_init_ws/2^20  rst=off  en=on  dbl_ovrd=off  block_type=register
  dx_A_o : Outport
  dy_A_o : Outport  Port=2
  dx_B_o : Outport  Port=3
  dy_B_o : Outport  Port=4
  wires:
  Convert7/1 -> Mux3/3
  Convert6/1 -> Mux3/2
  Convert5/1 -> Mux2/3
  Convert4/1 -> Mux2/2
  Convert3/1 -> Mux1/3
  Convert2/1 -> Mux1/2
  Convert1/1 -> Mux/3
  Convert/1 -> Mux/2
  dy_r/1 -> dy_pl_col_dely/2, dy_A_o/1
  Mux3/1 -> dy_r/1
  dy_pl_col_dely/1 -> Convert6/1
  dx_r/1 -> dx_pl_col_delx/1, dx_A_o/1
  Mux2/1 -> dx_r/1
  dx_pl_col_delx/1 -> Convert4/1
  ystart_r/1 -> Convert7/1, ystart_pl_row_deky/2
  Mux1/1 -> ystart_r/1
  ystart_pl_row_deky/1 -> Convert2/1
  xstart_r/1 -> Convert5/1, xstart_pl_row_delx/1
  Mux/1 -> xstart_r/1
  xstart_pl_row_delx/1 -> Convert/1
  der_i/1 -> Delay2/1
  fvf_i/1 -> Delay3/1, ystart_init/2, col_delx/2, col_dely1/2, col_delx1/2, ystart_init1/2, row_dely1/2, xstart_init1/2, row_delx1/2, col_dely/2, row_dely/2, xstart_init/2, row_delx/2
  ystart_init_A_i/1 -> ystart_init/1
  ystart_init/1 -> Reinterpret3/1
  row_dely/1 -> Reinterpret2/1, BitBasher1/1
  xstart_init/1 -> Reinterpret1/1
  row_delx/1 -> Reinterpret12/1, BitBasher2/1
  Delay2/1 -> Expression/2, Mux2/1, Mux3/1, Mux7/1, Mux6/1
  de_i/1 -> Delay5/1
  Delay5/1 -> dx_r/2, dy_r/2, dy_r1/2, dx_r1/2
  Delay3/1 -> Mux/1, Mux1/1, Mux5/1, Mux4/1, Expression/1
  Expression/1 -> xstart_r/2, ystart_r/2, ystart_r1/2, xstart_r1/2
  Reinterpret2/1 -> ystart_pl_row_deky/1
  Constant/1 -> row_delx_A_i/1, row_delx_B_i/1
  Constant1/1 -> xstart_init_A_i/1, xstart_init_B_i/1
  Constant2/1 -> row_dely_A_i/1, row_dely_B_i/1
  Constant3/1 -> ystart_init_A_i/1, ystart_init_B_i/1
  row_dely_A_i/1 -> row_dely/1
  xstart_init_A_i/1 -> xstart_init/1
  row_delx_A_i/1 -> row_delx/1
  Convert15/1 -> Mux7/3
  Convert14/1 -> Mux7/2
  Convert13/1 -> Mux6/3
  Convert12/1 -> Mux6/2
  Convert11/1 -> Mux5/3
  Convert10/1 -> Mux5/2
  Convert9/1 -> Mux4/3
  Convert8/1 -> Mux4/2
  dy_r1/1 -> dy_pl_col_dely1/2, dy_B_o/1
  Mux7/1 -> dy_r1/1
  dy_pl_col_dely1/1 -> Convert14/1
  dx_r1/1 -> dx_pl_col_delx1/1, dx_B_o/1
  Mux6/1 -> dx_r1/1
  dx_pl_col_delx1/1 -> Convert12/1
  ystart_r1/1 -> Convert15/1, ystart_pl_row_dely/2
  Mux5/1 -> ystart_r1/1
  ystart_pl_row_dely/1 -> Convert10/1
  xstart_r1/1 -> Convert13/1, xstart_pl_row_delx1/1
  Mux4/1 -> xstart_r1/1
  xstart_pl_row_delx1/1 -> Convert8/1
  ystart_init_B_i/1 -> ystart_init1/1
  ystart_init1/1 -> Reinterpret7/1
  row_dely1/1 -> Reinterpret6/1, BitBasher4/1
  xstart_init1/1 -> Reinterpret5/1
  row_delx1/1 -> Reinterpret4/1, BitBasher3/1
  Reinterpret4/1 -> xstart_pl_row_delx1/2
  Reinterpret6/1 -> ystart_pl_row_dely/1
  row_dely_B_i/1 -> row_dely1/1
  xstart_init_B_i/1 -> xstart_init1/1
  row_delx_B_i/1 -> row_delx1/1
  Constant8/1 -> col_delx_A_i/1, col_delx_B_i/1
  Constant9/1 -> col_dely_A_i/1, col_dely_B_i/1
  col_delx_A_i/1 -> col_delx/1
  col_dely_A_i/1 -> col_dely/1
  col_delx/1 -> Reinterpret8/1
  col_dely/1 -> Reinterpret9/1
  Reinterpret8/1 -> dx_pl_col_delx/2
  Reinterpret9/1 -> dy_pl_col_dely/1
  col_delx_B_i/1 -> col_delx1/1
  col_dely_B_i/1 -> col_dely1/1
  col_delx1/1 -> Reinterpret10/1
  col_dely1/1 -> Reinterpret11/1
  Reinterpret10/1 -> dx_pl_col_delx1/2
  Reinterpret11/1 -> dy_pl_col_dely1/1
  Mux8/1 -> Convert3/1
  Reinterpret3/1 -> y_start_i_pl_row_dely/1, Mux8/3
  Mux9/1 -> Convert1/1
  Reinterpret1/1 -> x_start_i_pl_row_delx/1, Mux9/3
  field_i/1 -> Delay1/1
  Delay1/1 -> Mux9/1, Mux8/1, Mux10/1, Mux11/1
  Mux10/1 -> Convert9/1
  Mux11/1 -> Convert11/1
  Reinterpret5/1 -> x_start_i_pl_row_delx1/1, Mux10/3
  Reinterpret7/1 -> x_start_i_pl_row_dely2/1, Mux11/3
  Reinterpret12/1 -> xstart_pl_row_delx/2
  BitBasher2/1 -> Reinterpret13/1
  Reinterpret13/1 -> x_start_i_pl_row_delx/2
  Reinterpret14/1 -> y_start_i_pl_row_dely/2
  BitBasher1/1 -> Reinterpret14/1
  BitBasher3/1 -> Reinterpret15/1
  Reinterpret15/1 -> x_start_i_pl_row_delx1/2
  BitBasher4/1 -> Reinterpret16/1
  Reinterpret16/1 -> x_start_i_pl_row_dely2/2
  y_start_i_pl_row_dely/1 -> Mux8/2
  x_start_i_pl_row_delx/1 -> Mux9/2
  x_start_i_pl_row_dely2/1 -> Mux11/2
  x_start_i_pl_row_delx1/1 -> Mux10/2

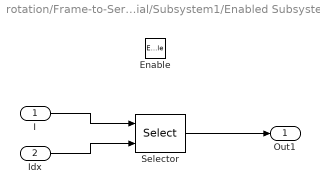
== system rotation/Frame-to-Serial/Subsystem1/Enabled Subsystem ==
  I : Inport  OutDataType=sfix(16)  OutScaling=2^0
  Idx : Inport  Port=2  OutDataType=sfix(16)  OutScaling=2^0
  Enable : EnablePort
  Selector : Selector  InputPortWidth=rows*cols  SampleTime=(1/fps)/(rows*(cols+2*blk))  IndexOptions=Index vector (port)  Indices=[1 4]  OutputSizes=1
  Out1 : Outport  OutDataType=sfix(16)  OutScaling=2^0
  wires:
  Selector/1 -> Out1/1
  I/1 -> Selector/1
  Idx/1 -> Selector/2
